simulink model "assemblage_19"  (R2016a)
settings: Solver=ode15s  StartTime=0.0  StopTime=1e6  RelTol=1e-3
undefined symbols (not defined in the file or in its folder): W
libraries: simCryogenics_lib x424, nesl_utility x343, fl_lib x9
(part 3 of 3)

== system assemblage_19/Cryomodules/CMB1 ==
  BP_out-E25 : simCryogenics_lib/Sensors/PTT
  BP_out-E26 : simCryogenics_lib/Sensors/PTT
  Bias25 : Bias  Bias=-50
  Bias26 : Bias  Bias=100
  Constant36 : Constant  Value=W
  Constant37 : Constant  Value=0
  Constant38 : Constant  Value=63
  Distributor19 : simCryogenics_lib/Elements/Distributor2
  FCV00 2 13 : simCryogenics_lib/Elements/Valve  CVmax=0.2  ControlInputMin=0  ControlInputMax=100  Xt=0.86  Rv=100  lin_v=0  lim_v=0  K=2.4e-5 m^1.50000*kg^0.50000/s/bar^0.50000  Cmd_specify=off  Cmd_priority=High  Cmd=0  gamma_specify=off  gamma_priority=High  gamma=0  rho_specify=off  rho_priority=High  rho=0 kg/m^3  Xc_specify=off  Xc_priority=High  Xc=0  X_specify=off  X_priority=High  X=0  Y_specify=off  Y_priority=High  Y=0  CV_specify=off  CV_priority=High  CV=0
  FCV25 : simCryogenics_lib/Elements/Valve  CVmax=1.25  ControlInputMin=0  ControlInputMax=100  Xt=0.86  Rv=150  lin_v=0  lim_v=0  K=2.4e-5 m^1.50000*kg^0.50000/s/bar^0.50000  Cmd_specify=off  Cmd_priority=High  Cmd=0  gamma_specify=off  gamma_priority=High  gamma=0  rho_specify=off  rho_priority=High  rho=0 kg/m^3  Xc_specify=off  Xc_priority=High  Xc=0  X_specify=off  X_priority=High  X=0  Y_specify=off  Y_priority=High  Y=0  CV_specify=off  CV_priority=High  CV=0
  FCV26 : simCryogenics_lib/Elements/Valve  CVmax=1.5  ControlInputMin=0  ControlInputMax=100  Xt=0.86  Rv=100  lin_v=0  lim_v=0  K=2.4e-5 m^1.50000*kg^0.50000/s/bar^0.50000  Cmd_specify=off  Cmd_priority=High  Cmd=0  gamma_specify=off  gamma_priority=High  gamma=0  rho_specify=off  rho_priority=High  rho=0 kg/m^3  Xc_specify=off  Xc_priority=High  Xc=0  X_specify=off  X_priority=High  X=0  Y_specify=off  Y_priority=High  Y=0  CV_specify=off  CV_priority=High  CV=0
  FT73 : simCryogenics_lib/Sensors/FT
  FT74 : Scope
  FT75 : Scope
  FT76 : simCryogenics_lib/Sensors/FT
  FT77 : simCryogenics_lib/Sensors/FT
  FT78 : Scope
  Gain13 : Gain  Gain=-10
  M src37 : simCryogenics_lib/Sources_Sinks/M src  M=0 kg/s
  M src38 : simCryogenics_lib/Sources_Sinks/M src  M=0 kg/s
  M src39 : simCryogenics_lib/Sources_Sinks/M src  M=0 kg/s
  Mixer21 : simCryogenics_lib/Elements/Mixer2
  Mux37 : Mux  Inputs=2
  Mux38 : Mux  Inputs=2
  Mux39 : Mux  Inputs=2
  P/T src25 : simCryogenics_lib/Sources_Sinks/P//T src  P=1.2 bar  T=4.4 K
  P/T src26 : simCryogenics_lib/Sources_Sinks/P//T src  P=1.2 bar  T=4.4 K
  PS-Simulink Converter{133..143} (11 alike) : nesl_utility/PS-Simulink Converter  PhysicalDomain=network_engine_domain  SubClassName=ps_output  LeftPortType=input  RightPortType=output  PseudoPeriodic=off  Frequencies=[]  Unit=1  AffineConversion=off
  PhaseSep13 : simCryogenics_lib/Elements/PhaseSep  Ideal1=1  DeltaT1=0.05 K  N1=10  h1=400 W/K  Ideal2=1  DeltaT2=0.05 K  N2=10  h2=400 W/K  hmax=0.870 m  S=0.0402 m^2  P0=1.25 bar  h0=50  T0=4.5 K
  Simulink-PS Converter{49..52} (4 alike) : nesl_utility/Simulink-PS Converter  PhysicalDomain=network_engine_domain  SubClassName=ps_input  LeftPortType=input  RightPortType=output  PseudoPeriodic=off  Frequencies=[]  NoiseDistribution=none  NoiseParameters=[]  Unit=1  AffineConversion=off  InputFiltering=off  SimscapeFilterOrder=1  InputFilterTimeConstant=0.001  UdotUserProvided=1
  TT49 : Scope
  TT50 : Scope
  TT51 : simCryogenics_lib/Sensors/PTT
  TT52 : Scope
  scope37 : Scope
  scope38 : Scope
  scope39 : Scope
  to_coldbox : PMIOPort  Port=1  Side=Left
  from_dewar : PMIOPort  Port=2  Side=Right
  wires:
  PS-Simulink Converter138/1 -> Mux38/1
  PS-Simulink Converter143/1 -> scope37/1
  Mux38/1 -> TT52/1
  PS-Simulink Converter133/1 -> FT78/1
  Bias26/1 -> scope38/1, Simulink-PS Converter51/1
  Mux37/1 -> TT49/1
  Bias25/1 -> Gain13/1
  Mux39/1 -> TT50/1
  Gain13/1 -> Bias26/1
  PS-Simulink Converter134/1 -> Mux39/1
  PS-Simulink Converter139/1 -> FT75/1
  Constant37/1 -> Simulink-PS Converter50/1
  PS-Simulink Converter137/1 -> FT74/1
  PS-Simulink Converter141/1 -> Mux38/2
  Constant38/1 -> Simulink-PS Converter52/1
  PS-Simulink Converter142/1 -> scope39/1, Bias25/1
  PS-Simulink Converter136/1 -> Mux37/2
  PS-Simulink Converter140/1 -> Mux37/1
  Constant36/1 -> Simulink-PS Converter49/1
  PS-Simulink Converter135/1 -> Mux39/2
  connections:
  Simulink-PS Converter51/RConn1 -- FCV25/LConn1
  BP_out-E26/RConn2 -- PS-Simulink Converter138/LConn1
  FCV26/LConn2 -- PhaseSep13/LConn1 -- BP_out-E25/LConn1 -- FT77/LConn1
  PS-Simulink Converter139/LConn1 -- FT77/RConn1
  PS-Simulink Converter137/LConn1 -- FT73/RConn1
  BP_out-E25/RConn1 -- PS-Simulink Converter135/LConn1
  Simulink-PS Converter50/RConn1 -- FCV00 2 13/LConn1
  PhaseSep13/LConn2 -- P/T src25/RConn1
  from_dewar/RConn1 -- Distributor19/LConn1
  M src37/RConn1 -- PhaseSep13/RConn1
  FCV26/LConn1 -- Simulink-PS Converter52/RConn1
  FCV00 2 13/LConn2 -- Distributor19/RConn1
  PhaseSep13/LConn4 -- Mixer21/RConn1
  FT73/LConn1 -- TT51/LConn1 -- FCV00 2 13/RConn1 -- Mixer21/LConn1
  BP_out-E25/RConn2 -- PS-Simulink Converter134/LConn1
  TT51/RConn1 -- PS-Simulink Converter140/LConn1
  PS-Simulink Converter142/LConn1 -- PhaseSep13/RConn5
  FCV25/RConn1 -- Mixer21/LConn2 -- FT76/LConn1 -- BP_out-E26/LConn1
  PS-Simulink Converter143/LConn1 -- PhaseSep13/LConn5
  M src39/RConn1 -- PhaseSep13/RConn3
  TT51/RConn2 -- PS-Simulink Converter136/LConn1
  FCV26/RConn1 -- to_coldbox/RConn1
  Distributor19/RConn2 -- FCV25/LConn2
  BP_out-E26/RConn1 -- PS-Simulink Converter141/LConn1
  PS-Simulink Converter133/LConn1 -- FT76/RConn1
  PhaseSep13/RConn2 -- M src38/RConn1
  P/T src26/RConn1 -- PhaseSep13/LConn3
  Simulink-PS Converter49/RConn1 -- PhaseSep13/RConn4

== system assemblage_19/Cryomodules/CMB2 ==
  BP_out-E27 : simCryogenics_lib/Sensors/PTT
  BP_out-E28 : simCryogenics_lib/Sensors/PTT
  Bias27 : Bias  Bias=-50
  Bias28 : Bias  Bias=100
  Constant39 : Constant  Value=W
  Constant40 : Constant  Value=0
  Constant41 : Constant  Value=63
  Distributor20 : simCryogenics_lib/Elements/Distributor2
  FCV00 2 14 : simCryogenics_lib/Elements/Valve  CVmax=0.2  ControlInputMin=0  ControlInputMax=100  Xt=0.86  Rv=100  lin_v=0  lim_v=0  K=2.4e-5 m^1.50000*kg^0.50000/s/bar^0.50000  Cmd_specify=off  Cmd_priority=High  Cmd=0  gamma_specify=off  gamma_priority=High  gamma=0  rho_specify=off  rho_priority=High  rho=0 kg/m^3  Xc_specify=off  Xc_priority=High  Xc=0  X_specify=off  X_priority=High  X=0  Y_specify=off  Y_priority=High  Y=0  CV_specify=off  CV_priority=High  CV=0
  FCV27 : simCryogenics_lib/Elements/Valve  CVmax=1.25  ControlInputMin=0  ControlInputMax=100  Xt=0.86  Rv=150  lin_v=0  lim_v=0  K=2.4e-5 m^1.50000*kg^0.50000/s/bar^0.50000  Cmd_specify=off  Cmd_priority=High  Cmd=0  gamma_specify=off  gamma_priority=High  gamma=0  rho_specify=off  rho_priority=High  rho=0 kg/m^3  Xc_specify=off  Xc_priority=High  Xc=0  X_specify=off  X_priority=High  X=0  Y_specify=off  Y_priority=High  Y=0  CV_specify=off  CV_priority=High  CV=0
  FCV28 : simCryogenics_lib/Elements/Valve  CVmax=1.5  ControlInputMin=0  ControlInputMax=100  Xt=0.86  Rv=100  lin_v=0  lim_v=0  K=2.4e-5 m^1.50000*kg^0.50000/s/bar^0.50000  Cmd_specify=off  Cmd_priority=High  Cmd=0  gamma_specify=off  gamma_priority=High  gamma=0  rho_specify=off  rho_priority=High  rho=0 kg/m^3  Xc_specify=off  Xc_priority=High  Xc=0  X_specify=off  X_priority=High  X=0  Y_specify=off  Y_priority=High  Y=0  CV_specify=off  CV_priority=High  CV=0
  FT79 : simCryogenics_lib/Sensors/FT
  FT80 : Scope
  FT81 : Scope
  FT82 : simCryogenics_lib/Sensors/FT
  FT83 : simCryogenics_lib/Sensors/FT
  FT84 : Scope
  Gain14 : Gain  Gain=-10
  M src40 : simCryogenics_lib/Sources_Sinks/M src  M=0 kg/s
  M src41 : simCryogenics_lib/Sources_Sinks/M src  M=0 kg/s
  M src42 : simCryogenics_lib/Sources_Sinks/M src  M=0 kg/s
  Mixer22 : simCryogenics_lib/Elements/Mixer2
  Mux40 : Mux  Inputs=2
  Mux41 : Mux  Inputs=2
  Mux42 : Mux  Inputs=2
  P/T src27 : simCryogenics_lib/Sources_Sinks/P//T src  P=1.2 bar  T=4.4 K
  P/T src28 : simCryogenics_lib/Sources_Sinks/P//T src  P=1.2 bar  T=4.4 K
  PS-Simulink Converter{144..154} (11 alike) : nesl_utility/PS-Simulink Converter  PhysicalDomain=network_engine_domain  SubClassName=ps_output  LeftPortType=input  RightPortType=output  PseudoPeriodic=off  Frequencies=[]  Unit=1  AffineConversion=off
  PhaseSep14 : simCryogenics_lib/Elements/PhaseSep  Ideal1=1  DeltaT1=0.05 K  N1=10  h1=400 W/K  Ideal2=1  DeltaT2=0.05 K  N2=10  h2=400 W/K  hmax=0.870 m  S=0.0402 m^2  P0=1.25 bar  h0=50  T0=4.5 K
  Simulink-PS Converter{53..56} (4 alike) : nesl_utility/Simulink-PS Converter  PhysicalDomain=network_engine_domain  SubClassName=ps_input  LeftPortType=input  RightPortType=output  PseudoPeriodic=off  Frequencies=[]  NoiseDistribution=none  NoiseParameters=[]  Unit=1  AffineConversion=off  InputFiltering=off  SimscapeFilterOrder=1  InputFilterTimeConstant=0.001  UdotUserProvided=1
  TT53 : Scope
  TT54 : Scope
  TT55 : simCryogenics_lib/Sensors/PTT
  TT56 : Scope
  scope40 : Scope
  scope41 : Scope
  scope42 : Scope
  to_coldbox : PMIOPort  Port=1  Side=Left
  from_dewar : PMIOPort  Port=2  Side=Right
  wires:
  PS-Simulink Converter149/1 -> Mux41/1
  PS-Simulink Converter148/1 -> FT80/1
  Mux40/1 -> TT53/1
  PS-Simulink Converter151/1 -> Mux40/1
  Bias28/1 -> scope41/1, Simulink-PS Converter55/1
  PS-Simulink Converter147/1 -> Mux40/2
  Constant40/1 -> Simulink-PS Converter54/1
  PS-Simulink Converter145/1 -> Mux42/1
  Constant39/1 -> Simulink-PS Converter53/1
  PS-Simulink Converter150/1 -> FT81/1
  Mux42/1 -> TT54/1
  Gain14/1 -> Bias28/1
  PS-Simulink Converter144/1 -> FT84/1
  PS-Simulink Converter146/1 -> Mux42/2
  Bias27/1 -> Gain14/1
  Constant41/1 -> Simulink-PS Converter56/1
  PS-Simulink Converter152/1 -> Mux41/2
  PS-Simulink Converter154/1 -> scope40/1
  Mux41/1 -> TT56/1
  PS-Simulink Converter153/1 -> scope42/1, Bias27/1
  connections:
  FCV28/LConn2 -- PhaseSep14/LConn1 -- BP_out-E27/LConn1 -- FT83/LConn1
  FT79/LConn1 -- TT55/LConn1 -- FCV00 2 14/RConn1 -- Mixer22/LConn1
  BP_out-E27/RConn1 -- PS-Simulink Converter146/LConn1
  Distributor20/RConn2 -- FCV27/LConn2
  PS-Simulink Converter154/LConn1 -- PhaseSep14/LConn5
  BP_out-E28/RConn1 -- PS-Simulink Converter152/LConn1
  Simulink-PS Converter54/RConn1 -- FCV00 2 14/LConn1
  PhaseSep14/RConn2 -- M src41/RConn1
  TT55/RConn1 -- PS-Simulink Converter151/LConn1
  BP_out-E28/RConn2 -- PS-Simulink Converter149/LConn1
  FCV28/LConn1 -- Simulink-PS Converter56/RConn1
  PS-Simulink Converter153/LConn1 -- PhaseSep14/RConn5
  from_dewar/RConn1 -- Distributor20/LConn1
  M src42/RConn1 -- PhaseSep14/RConn3
  TT55/RConn2 -- PS-Simulink Converter147/LConn1
  PhaseSep14/LConn2 -- P/T src27/RConn1
  FCV28/RConn1 -- to_coldbox/RConn1
  P/T src28/RConn1 -- PhaseSep14/LConn3
  BP_out-E27/RConn2 -- PS-Simulink Converter145/LConn1
  FCV00 2 14/LConn2 -- Distributor20/RConn1
  PS-Simulink Converter144/LConn1 -- FT82/RConn1
  Simulink-PS Converter53/RConn1 -- PhaseSep14/RConn4
  Simulink-PS Converter55/RConn1 -- FCV27/LConn1
  PS-Simulink Converter148/LConn1 -- FT79/RConn1
  PhaseSep14/LConn4 -- Mixer22/RConn1
  PS-Simulink Converter150/LConn1 -- FT83/RConn1
  FCV27/RConn1 -- Mixer22/LConn2 -- FT82/LConn1 -- BP_out-E28/LConn1
  M src40/RConn1 -- PhaseSep14/RConn1

== system assemblage_19/Cryomodules/CMB3 ==
  BP_out-E29 : simCryogenics_lib/Sensors/PTT
  BP_out-E30 : simCryogenics_lib/Sensors/PTT
  Bias29 : Bias  Bias=-50
  Bias30 : Bias  Bias=100
  Constant42 : Constant  Value=W
  Constant43 : Constant  Value=0
  Constant44 : Constant  Value=63
  Distributor21 : simCryogenics_lib/Elements/Distributor2
  FCV00 2 15 : simCryogenics_lib/Elements/Valve  CVmax=0.2  ControlInputMin=0  ControlInputMax=100  Xt=0.86  Rv=100  lin_v=0  lim_v=0  K=2.4e-5 m^1.50000*kg^0.50000/s/bar^0.50000  Cmd_specify=off  Cmd_priority=High  Cmd=0  gamma_specify=off  gamma_priority=High  gamma=0  rho_specify=off  rho_priority=High  rho=0 kg/m^3  Xc_specify=off  Xc_priority=High  Xc=0  X_specify=off  X_priority=High  X=0  Y_specify=off  Y_priority=High  Y=0  CV_specify=off  CV_priority=High  CV=0
  FCV29 : simCryogenics_lib/Elements/Valve  CVmax=1.25  ControlInputMin=0  ControlInputMax=100  Xt=0.86  Rv=150  lin_v=0  lim_v=0  K=2.4e-5 m^1.50000*kg^0.50000/s/bar^0.50000  Cmd_specify=off  Cmd_priority=High  Cmd=0  gamma_specify=off  gamma_priority=High  gamma=0  rho_specify=off  rho_priority=High  rho=0 kg/m^3  Xc_specify=off  Xc_priority=High  Xc=0  X_specify=off  X_priority=High  X=0  Y_specify=off  Y_priority=High  Y=0  CV_specify=off  CV_priority=High  CV=0
  FCV30 : simCryogenics_lib/Elements/Valve  CVmax=1.5  ControlInputMin=0  ControlInputMax=100  Xt=0.86  Rv=100  lin_v=0  lim_v=0  K=2.4e-5 m^1.50000*kg^0.50000/s/bar^0.50000  Cmd_specify=off  Cmd_priority=High  Cmd=0  gamma_specify=off  gamma_priority=High  gamma=0  rho_specify=off  rho_priority=High  rho=0 kg/m^3  Xc_specify=off  Xc_priority=High  Xc=0  X_specify=off  X_priority=High  X=0  Y_specify=off  Y_priority=High  Y=0  CV_specify=off  CV_priority=High  CV=0
  FT85 : simCryogenics_lib/Sensors/FT
  FT86 : Scope
  FT87 : Scope
  FT88 : simCryogenics_lib/Sensors/FT
  FT89 : simCryogenics_lib/Sensors/FT
  FT90 : Scope
  Gain15 : Gain  Gain=-10
  M src43 : simCryogenics_lib/Sources_Sinks/M src  M=0 kg/s
  M src44 : simCryogenics_lib/Sources_Sinks/M src  M=0 kg/s
  M src45 : simCryogenics_lib/Sources_Sinks/M src  M=0 kg/s
  Mixer23 : simCryogenics_lib/Elements/Mixer2
  Mux43 : Mux  Inputs=2
  Mux44 : Mux  Inputs=2
  Mux45 : Mux  Inputs=2
  P/T src29 : simCryogenics_lib/Sources_Sinks/P//T src  P=1.2 bar  T=4.4 K
  P/T src30 : simCryogenics_lib/Sources_Sinks/P//T src  P=1.2 bar  T=4.4 K
  PS-Simulink Converter{155..165} (11 alike) : nesl_utility/PS-Simulink Converter  PhysicalDomain=network_engine_domain  SubClassName=ps_output  LeftPortType=input  RightPortType=output  PseudoPeriodic=off  Frequencies=[]  Unit=1  AffineConversion=off
  PhaseSep15 : simCryogenics_lib/Elements/PhaseSep  Ideal1=1  DeltaT1=0.05 K  N1=10  h1=400 W/K  Ideal2=1  DeltaT2=0.05 K  N2=10  h2=400 W/K  hmax=0.870 m  S=0.0402 m^2  P0=1.25 bar  h0=50  T0=4.5 K
  Simulink-PS Converter{57..60} (4 alike) : nesl_utility/Simulink-PS Converter  PhysicalDomain=network_engine_domain  SubClassName=ps_input  LeftPortType=input  RightPortType=output  PseudoPeriodic=off  Frequencies=[]  NoiseDistribution=none  NoiseParameters=[]  Unit=1  AffineConversion=off  InputFiltering=off  SimscapeFilterOrder=1  InputFilterTimeConstant=0.001  UdotUserProvided=1
  TT57 : Scope
  TT58 : Scope
  TT59 : simCryogenics_lib/Sensors/PTT
  TT60 : Scope
  scope43 : Scope
  scope44 : Scope
  scope45 : Scope
  to_coldbox : PMIOPort  Port=1  Side=Left
  from_dewar : PMIOPort  Port=2  Side=Right
  wires:
  Bias29/1 -> Gain15/1
  PS-Simulink Converter160/1 -> Mux44/1
  Constant43/1 -> Simulink-PS Converter58/1
  PS-Simulink Converter161/1 -> FT87/1
  PS-Simulink Converter157/1 -> Mux45/2
  Constant42/1 -> Simulink-PS Converter57/1
  PS-Simulink Converter159/1 -> FT86/1
  Mux44/1 -> TT60/1
  PS-Simulink Converter164/1 -> scope45/1, Bias29/1
  PS-Simulink Converter163/1 -> Mux44/2
  Constant44/1 -> Simulink-PS Converter60/1
  Gain15/1 -> Bias30/1
  PS-Simulink Converter155/1 -> FT90/1
  PS-Simulink Converter165/1 -> scope43/1
  PS-Simulink Converter156/1 -> Mux45/1
  Mux43/1 -> TT57/1
  PS-Simulink Converter162/1 -> Mux43/1
  Bias30/1 -> scope44/1, Simulink-PS Converter59/1
  Mux45/1 -> TT58/1
  PS-Simulink Converter158/1 -> Mux43/2
  connections:
  PS-Simulink Converter155/LConn1 -- FT88/RConn1
  FT85/LConn1 -- TT59/LConn1 -- FCV00 2 15/RConn1 -- Mixer23/LConn1
  BP_out-E29/RConn2 -- PS-Simulink Converter156/LConn1
  P/T src30/RConn1 -- PhaseSep15/LConn3
  PS-Simulink Converter159/LConn1 -- FT85/RConn1
  M src43/RConn1 -- PhaseSep15/RConn1
  M src45/RConn1 -- PhaseSep15/RConn3
  BP_out-E30/RConn1 -- PS-Simulink Converter163/LConn1
  BP_out-E30/RConn2 -- PS-Simulink Converter160/LConn1
  PS-Simulink Converter164/LConn1 -- PhaseSep15/RConn5
  PS-Simulink Converter165/LConn1 -- PhaseSep15/LConn5
  BP_out-E29/RConn1 -- PS-Simulink Converter157/LConn1
  from_dewar/RConn1 -- Distributor21/LConn1
  PhaseSep15/LConn4 -- Mixer23/RConn1
  TT59/RConn1 -- PS-Simulink Converter162/LConn1
  FCV00 2 15/LConn2 -- Distributor21/RConn1
  Simulink-PS Converter58/RConn1 -- FCV00 2 15/LConn1
  PhaseSep15/RConn2 -- M src44/RConn1
  Simulink-PS Converter59/RConn1 -- FCV29/LConn1
  Distributor21/RConn2 -- FCV29/LConn2
  TT59/RConn2 -- PS-Simulink Converter158/LConn1
  FCV29/RConn1 -- Mixer23/LConn2 -- FT88/LConn1 -- BP_out-E30/LConn1
  PS-Simulink Converter161/LConn1 -- FT89/RConn1
  Simulink-PS Converter57/RConn1 -- PhaseSep15/RConn4
  FCV30/RConn1 -- to_coldbox/RConn1
  PhaseSep15/LConn2 -- P/T src29/RConn1
  FCV30/LConn2 -- PhaseSep15/LConn1 -- BP_out-E29/LConn1 -- FT89/LConn1
  FCV30/LConn1 -- Simulink-PS Converter60/RConn1

== system assemblage_19/Cryomodules/CMB4 ==
  BP_out-E31 : simCryogenics_lib/Sensors/PTT
  BP_out-E32 : simCryogenics_lib/Sensors/PTT
  Bias31 : Bias  Bias=-50
  Bias32 : Bias  Bias=100
  Constant45 : Constant  Value=W
  Constant46 : Constant  Value=0
  Constant47 : Constant  Value=63
  Distributor22 : simCryogenics_lib/Elements/Distributor2
  FCV00 2 16 : simCryogenics_lib/Elements/Valve  CVmax=0.2  ControlInputMin=0  ControlInputMax=100  Xt=0.86  Rv=100  lin_v=0  lim_v=0  K=2.4e-5 m^1.50000*kg^0.50000/s/bar^0.50000  Cmd_specify=off  Cmd_priority=High  Cmd=0  gamma_specify=off  gamma_priority=High  gamma=0  rho_specify=off  rho_priority=High  rho=0 kg/m^3  Xc_specify=off  Xc_priority=High  Xc=0  X_specify=off  X_priority=High  X=0  Y_specify=off  Y_priority=High  Y=0  CV_specify=off  CV_priority=High  CV=0
  FCV31 : simCryogenics_lib/Elements/Valve  CVmax=1.25  ControlInputMin=0  ControlInputMax=100  Xt=0.86  Rv=150  lin_v=0  lim_v=0  K=2.4e-5 m^1.50000*kg^0.50000/s/bar^0.50000  Cmd_specify=off  Cmd_priority=High  Cmd=0  gamma_specify=off  gamma_priority=High  gamma=0  rho_specify=off  rho_priority=High  rho=0 kg/m^3  Xc_specify=off  Xc_priority=High  Xc=0  X_specify=off  X_priority=High  X=0  Y_specify=off  Y_priority=High  Y=0  CV_specify=off  CV_priority=High  CV=0
  FCV32 : simCryogenics_lib/Elements/Valve  CVmax=1.5  ControlInputMin=0  ControlInputMax=100  Xt=0.86  Rv=100  lin_v=0  lim_v=0  K=2.4e-5 m^1.50000*kg^0.50000/s/bar^0.50000  Cmd_specify=off  Cmd_priority=High  Cmd=0  gamma_specify=off  gamma_priority=High  gamma=0  rho_specify=off  rho_priority=High  rho=0 kg/m^3  Xc_specify=off  Xc_priority=High  Xc=0  X_specify=off  X_priority=High  X=0  Y_specify=off  Y_priority=High  Y=0  CV_specify=off  CV_priority=High  CV=0
  FT91 : simCryogenics_lib/Sensors/FT
  FT92 : Scope
  FT93 : Scope
  FT94 : simCryogenics_lib/Sensors/FT
  FT95 : simCryogenics_lib/Sensors/FT
  FT96 : Scope
  Gain16 : Gain  Gain=-10
  M src46 : simCryogenics_lib/Sources_Sinks/M src  M=0 kg/s
  M src47 : simCryogenics_lib/Sources_Sinks/M src  M=0 kg/s
  M src48 : simCryogenics_lib/Sources_Sinks/M src  M=0 kg/s
  Mixer24 : simCryogenics_lib/Elements/Mixer2
  Mux46 : Mux  Inputs=2
  Mux47 : Mux  Inputs=2
  Mux48 : Mux  Inputs=2
  P/T src31 : simCryogenics_lib/Sources_Sinks/P//T src  P=1.2 bar  T=4.4 K
  P/T src32 : simCryogenics_lib/Sources_Sinks/P//T src  P=1.2 bar  T=4.4 K
  PS-Simulink Converter{166..176} (11 alike) : nesl_utility/PS-Simulink Converter  PhysicalDomain=network_engine_domain  SubClassName=ps_output  LeftPortType=input  RightPortType=output  PseudoPeriodic=off  Frequencies=[]  Unit=1  AffineConversion=off
  PhaseSep16 : simCryogenics_lib/Elements/PhaseSep  Ideal1=1  DeltaT1=0.05 K  N1=10  h1=400 W/K  Ideal2=1  DeltaT2=0.05 K  N2=10  h2=400 W/K  hmax=0.870 m  S=0.0402 m^2  P0=1.25 bar  h0=50  T0=4.5 K
  Simulink-PS Converter{61..64} (4 alike) : nesl_utility/Simulink-PS Converter  PhysicalDomain=network_engine_domain  SubClassName=ps_input  LeftPortType=input  RightPortType=output  PseudoPeriodic=off  Frequencies=[]  NoiseDistribution=none  NoiseParameters=[]  Unit=1  AffineConversion=off  InputFiltering=off  SimscapeFilterOrder=1  InputFilterTimeConstant=0.001  UdotUserProvided=1
  TT61 : Scope
  TT62 : Scope
  TT63 : simCryogenics_lib/Sensors/PTT
  TT64 : Scope
  scope46 : Scope
  scope47 : Scope
  scope48 : Scope
  to_coldbox : PMIOPort  Port=1  Side=Left
  from_dewar : PMIOPort  Port=2  Side=Right
  wires:
  Gain16/1 -> Bias32/1
  PS-Simulink Converter173/1 -> Mux46/1
  PS-Simulink Converter166/1 -> FT96/1
  PS-Simulink Converter169/1 -> Mux46/2
  PS-Simulink Converter170/1 -> FT92/1
  Constant47/1 -> Simulink-PS Converter64/1
  PS-Simulink Converter171/1 -> Mux47/1
  PS-Simulink Converter176/1 -> scope46/1
  PS-Simulink Converter175/1 -> scope48/1, Bias31/1
  Mux48/1 -> TT62/1
  PS-Simulink Converter168/1 -> Mux48/2
  Constant45/1 -> Simulink-PS Converter61/1
  PS-Simulink Converter174/1 -> Mux47/2
  Bias31/1 -> Gain16/1
  Bias32/1 -> scope47/1, Simulink-PS Converter63/1
  PS-Simulink Converter167/1 -> Mux48/1
  Mux46/1 -> TT61/1
  Constant46/1 -> Simulink-PS Converter62/1
  PS-Simulink Converter172/1 -> FT93/1
  Mux47/1 -> TT64/1
  connections:
  PS-Simulink Converter170/LConn1 -- FT91/RConn1
  PS-Simulink Converter176/LConn1 -- PhaseSep16/LConn5
  Simulink-PS Converter61/RConn1 -- PhaseSep16/RConn4
  PS-Simulink Converter175/LConn1 -- PhaseSep16/RConn5
  BP_out-E31/RConn2 -- PS-Simulink Converter167/LConn1
  M src48/RConn1 -- PhaseSep16/RConn3
  P/T src32/RConn1 -- PhaseSep16/LConn3
  PhaseSep16/LConn4 -- Mixer24/RConn1
  PhaseSep16/LConn2 -- P/T src31/RConn1
  FT91/LConn1 -- TT63/LConn1 -- FCV00 2 16/RConn1 -- Mixer24/LConn1
  BP_out-E31/RConn1 -- PS-Simulink Converter168/LConn1
  Simulink-PS Converter62/RConn1 -- FCV00 2 16/LConn1
  BP_out-E32/RConn1 -- PS-Simulink Converter174/LConn1
  M src46/RConn1 -- PhaseSep16/RConn1
  TT63/RConn1 -- PS-Simulink Converter173/LConn1
  FCV32/LConn1 -- Simulink-PS Converter64/RConn1
  FCV31/RConn1 -- Mixer24/LConn2 -- FT94/LConn1 -- BP_out-E32/LConn1
  FCV32/RConn1 -- to_coldbox/RConn1
  FCV00 2 16/LConn2 -- Distributor22/RConn1
  PS-Simulink Converter172/LConn1 -- FT95/RConn1
  PS-Simulink Converter166/LConn1 -- FT94/RConn1
  Simulink-PS Converter63/RConn1 -- FCV31/LConn1
  PhaseSep16/RConn2 -- M src47/RConn1
  Distributor22/RConn2 -- FCV31/LConn2
  from_dewar/RConn1 -- Distributor22/LConn1
  TT63/RConn2 -- PS-Simulink Converter169/LConn1
  FCV32/LConn2 -- PhaseSep16/LConn1 -- BP_out-E31/LConn1 -- FT95/LConn1
  BP_out-E32/RConn2 -- PS-Simulink Converter171/LConn1

== system assemblage_19/Cryomodules/CMB5 ==
  BP_out-E33 : simCryogenics_lib/Sensors/PTT
  BP_out-E34 : simCryogenics_lib/Sensors/PTT
  Bias33 : Bias  Bias=-50
  Bias34 : Bias  Bias=100
  Constant48 : Constant  Value=W
  Constant49 : Constant  Value=0
  Constant50 : Constant  Value=63
  Distributor23 : simCryogenics_lib/Elements/Distributor2
  FCV00 2 17 : simCryogenics_lib/Elements/Valve  CVmax=0.2  ControlInputMin=0  ControlInputMax=100  Xt=0.86  Rv=100  lin_v=0  lim_v=0  K=2.4e-5 m^1.50000*kg^0.50000/s/bar^0.50000  Cmd_specify=off  Cmd_priority=High  Cmd=0  gamma_specify=off  gamma_priority=High  gamma=0  rho_specify=off  rho_priority=High  rho=0 kg/m^3  Xc_specify=off  Xc_priority=High  Xc=0  X_specify=off  X_priority=High  X=0  Y_specify=off  Y_priority=High  Y=0  CV_specify=off  CV_priority=High  CV=0
  FCV33 : simCryogenics_lib/Elements/Valve  CVmax=1.25  ControlInputMin=0  ControlInputMax=100  Xt=0.86  Rv=150  lin_v=0  lim_v=0  K=2.4e-5 m^1.50000*kg^0.50000/s/bar^0.50000  Cmd_specify=off  Cmd_priority=High  Cmd=0  gamma_specify=off  gamma_priority=High  gamma=0  rho_specify=off  rho_priority=High  rho=0 kg/m^3  Xc_specify=off  Xc_priority=High  Xc=0  X_specify=off  X_priority=High  X=0  Y_specify=off  Y_priority=High  Y=0  CV_specify=off  CV_priority=High  CV=0
  FCV34 : simCryogenics_lib/Elements/Valve  CVmax=1.5  ControlInputMin=0  ControlInputMax=100  Xt=0.86  Rv=100  lin_v=0  lim_v=0  K=2.4e-5 m^1.50000*kg^0.50000/s/bar^0.50000  Cmd_specify=off  Cmd_priority=High  Cmd=0  gamma_specify=off  gamma_priority=High  gamma=0  rho_specify=off  rho_priority=High  rho=0 kg/m^3  Xc_specify=off  Xc_priority=High  Xc=0  X_specify=off  X_priority=High  X=0  Y_specify=off  Y_priority=High  Y=0  CV_specify=off  CV_priority=High  CV=0
  FT100 : simCryogenics_lib/Sensors/FT
  FT101 : simCryogenics_lib/Sensors/FT
  FT102 : Scope
  FT97 : simCryogenics_lib/Sensors/FT
  FT98 : Scope
  FT99 : Scope
  Gain17 : Gain  Gain=-10
  M src49 : simCryogenics_lib/Sources_Sinks/M src  M=0 kg/s
  M src50 : simCryogenics_lib/Sources_Sinks/M src  M=0 kg/s
  M src51 : simCryogenics_lib/Sources_Sinks/M src  M=0 kg/s
  Mixer25 : simCryogenics_lib/Elements/Mixer2
  Mux49 : Mux  Inputs=2
  Mux50 : Mux  Inputs=2
  Mux51 : Mux  Inputs=2
  P/T src33 : simCryogenics_lib/Sources_Sinks/P//T src  P=1.2 bar  T=4.4 K
  P/T src34 : simCryogenics_lib/Sources_Sinks/P//T src  P=1.2 bar  T=4.4 K
  PS-Simulink Converter{177..187} (11 alike) : nesl_utility/PS-Simulink Converter  PhysicalDomain=network_engine_domain  SubClassName=ps_output  LeftPortType=input  RightPortType=output  PseudoPeriodic=off  Frequencies=[]  Unit=1  AffineConversion=off
  PhaseSep17 : simCryogenics_lib/Elements/PhaseSep  Ideal1=1  DeltaT1=0.05 K  N1=10  h1=400 W/K  Ideal2=1  DeltaT2=0.05 K  N2=10  h2=400 W/K  hmax=0.870 m  S=0.0402 m^2  P0=1.25 bar  h0=50  T0=4.5 K
  Simulink-PS Converter{65..68} (4 alike) : nesl_utility/Simulink-PS Converter  PhysicalDomain=network_engine_domain  SubClassName=ps_input  LeftPortType=input  RightPortType=output  PseudoPeriodic=off  Frequencies=[]  NoiseDistribution=none  NoiseParameters=[]  Unit=1  AffineConversion=off  InputFiltering=off  SimscapeFilterOrder=1  InputFilterTimeConstant=0.001  UdotUserProvided=1
  TT65 : Scope
  TT66 : Scope
  TT67 : simCryogenics_lib/Sensors/PTT
  TT68 : Scope
  scope49 : Scope
  scope50 : Scope
  scope51 : Scope
  to_coldbox : PMIOPort  Port=1  Side=Left
  from_dewar : PMIOPort  Port=2  Side=Right
  wires:
  PS-Simulink Converter186/1 -> scope51/1, Bias33/1
  PS-Simulink Converter187/1 -> scope49/1
  PS-Simulink Converter183/1 -> FT99/1
  Bias33/1 -> Gain17/1
  PS-Simulink Converter181/1 -> FT98/1
  Gain17/1 -> Bias34/1
  Constant49/1 -> Simulink-PS Converter66/1
  Mux50/1 -> TT68/1
  Mux51/1 -> TT66/1
  Constant50/1 -> Simulink-PS Converter68/1
  PS-Simulink Converter182/1 -> Mux50/1
  PS-Simulink Converter178/1 -> Mux51/1
  Constant48/1 -> Simulink-PS Converter65/1
  PS-Simulink Converter184/1 -> Mux49/1
  PS-Simulink Converter185/1 -> Mux50/2
  PS-Simulink Converter180/1 -> Mux49/2
  Bias34/1 -> scope50/1, Simulink-PS Converter67/1
  Mux49/1 -> TT65/1
  PS-Simulink Converter177/1 -> FT102/1
  PS-Simulink Converter179/1 -> Mux51/2
  connections:
  PhaseSep17/LConn2 -- P/T src33/RConn1
  FCV34/LConn1 -- Simulink-PS Converter68/RConn1
  FCV00 2 17/LConn2 -- Distributor23/RConn1
  Simulink-PS Converter67/RConn1 -- FCV33/LConn1
  PhaseSep17/LConn4 -- Mixer25/RConn1
  PS-Simulink Converter181/LConn1 -- FT97/RConn1
  Simulink-PS Converter65/RConn1 -- PhaseSep17/RConn4
  PS-Simulink Converter183/LConn1 -- FT101/RConn1
  M src49/RConn1 -- PhaseSep17/RConn1
  Simulink-PS Converter66/RConn1 -- FCV00 2 17/LConn1
  PhaseSep17/RConn2 -- M src50/RConn1
  BP_out-E34/RConn2 -- PS-Simulink Converter182/LConn1
  PS-Simulink Converter187/LConn1 -- PhaseSep17/LConn5
  M src51/RConn1 -- PhaseSep17/RConn3
  BP_out-E33/RConn1 -- PS-Simulink Converter179/LConn1
  PS-Simulink Converter186/LConn1 -- PhaseSep17/RConn5
  FCV34/LConn2 -- PhaseSep17/LConn1 -- BP_out-E33/LConn1 -- FT101/LConn1
  FCV34/RConn1 -- to_coldbox/RConn1
  PS-Simulink Converter177/LConn1 -- FT100/RConn1
  BP_out-E33/RConn2 -- PS-Simulink Converter178/LConn1
  BP_out-E34/RConn1 -- PS-Simulink Converter185/LConn1
  TT67/RConn2 -- PS-Simulink Converter180/LConn1
  P/T src34/RConn1 -- PhaseSep17/LConn3
  TT67/RConn1 -- PS-Simulink Converter184/LConn1
  from_dewar/RConn1 -- Distributor23/LConn1
  Distributor23/RConn2 -- FCV33/LConn2
  FT97/LConn1 -- TT67/LConn1 -- FCV00 2 17/RConn1 -- Mixer25/LConn1
  FCV33/RConn1 -- Mixer25/LConn2 -- FT100/LConn1 -- BP_out-E34/LConn1

== system assemblage_19/Cryomodules/CMB6 ==
  BP_out-E35 : simCryogenics_lib/Sensors/PTT
  BP_out-E36 : simCryogenics_lib/Sensors/PTT
  Bias35 : Bias  Bias=-50
  Bias36 : Bias  Bias=100
  Constant51 : Constant  Value=W
  Constant52 : Constant  Value=0
  Constant53 : Constant  Value=63
  Distributor24 : simCryogenics_lib/Elements/Distributor2
  FCV00 2 18 : simCryogenics_lib/Elements/Valve  CVmax=0.2  ControlInputMin=0  ControlInputMax=100  Xt=0.86  Rv=100  lin_v=0  lim_v=0  K=2.4e-5 m^1.50000*kg^0.50000/s/bar^0.50000  Cmd_specify=off  Cmd_priority=High  Cmd=0  gamma_specify=off  gamma_priority=High  gamma=0  rho_specify=off  rho_priority=High  rho=0 kg/m^3  Xc_specify=off  Xc_priority=High  Xc=0  X_specify=off  X_priority=High  X=0  Y_specify=off  Y_priority=High  Y=0  CV_specify=off  CV_priority=High  CV=0
  FCV35 : simCryogenics_lib/Elements/Valve  CVmax=1.25  ControlInputMin=0  ControlInputMax=100  Xt=0.86  Rv=150  lin_v=0  lim_v=0  K=2.4e-5 m^1.50000*kg^0.50000/s/bar^0.50000  Cmd_specify=off  Cmd_priority=High  Cmd=0  gamma_specify=off  gamma_priority=High  gamma=0  rho_specify=off  rho_priority=High  rho=0 kg/m^3  Xc_specify=off  Xc_priority=High  Xc=0  X_specify=off  X_priority=High  X=0  Y_specify=off  Y_priority=High  Y=0  CV_specify=off  CV_priority=High  CV=0
  FCV36 : simCryogenics_lib/Elements/Valve  CVmax=1.5  ControlInputMin=0  ControlInputMax=100  Xt=0.86  Rv=100  lin_v=0  lim_v=0  K=2.4e-5 m^1.50000*kg^0.50000/s/bar^0.50000  Cmd_specify=off  Cmd_priority=High  Cmd=0  gamma_specify=off  gamma_priority=High  gamma=0  rho_specify=off  rho_priority=High  rho=0 kg/m^3  Xc_specify=off  Xc_priority=High  Xc=0  X_specify=off  X_priority=High  X=0  Y_specify=off  Y_priority=High  Y=0  CV_specify=off  CV_priority=High  CV=0
  FT103 : simCryogenics_lib/Sensors/FT
  FT104 : Scope
  FT105 : Scope
  FT106 : simCryogenics_lib/Sensors/FT
  FT107 : simCryogenics_lib/Sensors/FT
  FT108 : Scope
  Gain18 : Gain  Gain=-10
  M src52 : simCryogenics_lib/Sources_Sinks/M src  M=0 kg/s
  M src53 : simCryogenics_lib/Sources_Sinks/M src  M=0 kg/s
  M src54 : simCryogenics_lib/Sources_Sinks/M src  M=0 kg/s
  Mixer26 : simCryogenics_lib/Elements/Mixer2
  Mux52 : Mux  Inputs=2
  Mux53 : Mux  Inputs=2
  Mux54 : Mux  Inputs=2
  P/T src35 : simCryogenics_lib/Sources_Sinks/P//T src  P=1.2 bar  T=4.4 K
  P/T src36 : simCryogenics_lib/Sources_Sinks/P//T src  P=1.2 bar  T=4.4 K
  PS-Simulink Converter{188..198} (11 alike) : nesl_utility/PS-Simulink Converter  PhysicalDomain=network_engine_domain  SubClassName=ps_output  LeftPortType=input  RightPortType=output  PseudoPeriodic=off  Frequencies=[]  Unit=1  AffineConversion=off
  PhaseSep18 : simCryogenics_lib/Elements/PhaseSep  Ideal1=1  DeltaT1=0.05 K  N1=10  h1=400 W/K  Ideal2=1  DeltaT2=0.05 K  N2=10  h2=400 W/K  hmax=0.870 m  S=0.0402 m^2  P0=1.25 bar  h0=50  T0=4.5 K
  Simulink-PS Converter{69..72} (4 alike) : nesl_utility/Simulink-PS Converter  PhysicalDomain=network_engine_domain  SubClassName=ps_input  LeftPortType=input  RightPortType=output  PseudoPeriodic=off  Frequencies=[]  NoiseDistribution=none  NoiseParameters=[]  Unit=1  AffineConversion=off  InputFiltering=off  SimscapeFilterOrder=1  InputFilterTimeConstant=0.001  UdotUserProvided=1
  TT69 : Scope
  TT70 : Scope
  TT71 : simCryogenics_lib/Sensors/PTT
  TT72 : Scope
  scope52 : Scope
  scope53 : Scope
  scope54 : Scope
  to_coldbox : PMIOPort  Port=1  Side=Left
  from_dewar : PMIOPort  Port=2  Side=Right
  wires:
  Mux52/1 -> TT69/1
  PS-Simulink Converter198/1 -> scope52/1
  PS-Simulink Converter196/1 -> Mux53/2
  PS-Simulink Converter189/1 -> Mux54/1
  Bias36/1 -> scope53/1, Simulink-PS Converter71/1
  Gain18/1 -> Bias36/1
  PS-Simulink Converter190/1 -> Mux54/2
  Constant53/1 -> Simulink-PS Converter72/1
  PS-Simulink Converter191/1 -> Mux52/2
  PS-Simulink Converter195/1 -> Mux52/1
  Bias35/1 -> Gain18/1
  PS-Simulink Converter197/1 -> scope54/1, Bias35/1
  PS-Simulink Converter193/1 -> Mux53/1
  PS-Simulink Converter194/1 -> FT105/1
  Constant51/1 -> Simulink-PS Converter69/1
  Mux54/1 -> TT70/1
  Mux53/1 -> TT72/1
  PS-Simulink Converter192/1 -> FT104/1
  PS-Simulink Converter188/1 -> FT108/1
  Constant52/1 -> Simulink-PS Converter70/1
  connections:
  FCV36/RConn1 -- to_coldbox/RConn1
  FCV36/LConn1 -- Simulink-PS Converter72/RConn1
  PS-Simulink Converter198/LConn1 -- PhaseSep18/LConn5
  Distributor24/RConn2 -- FCV35/LConn2
  P/T src36/RConn1 -- PhaseSep18/LConn3
  TT71/RConn2 -- PS-Simulink Converter191/LConn1
  FCV00 2 18/LConn2 -- Distributor24/RConn1
  PS-Simulink Converter197/LConn1 -- PhaseSep18/RConn5
  Simulink-PS Converter70/RConn1 -- FCV00 2 18/LConn1
  BP_out-E36/RConn2 -- PS-Simulink Converter193/LConn1
  PS-Simulink Converter188/LConn1 -- FT106/RConn1
  PhaseSep18/RConn2 -- M src53/RConn1
  PS-Simulink Converter192/LConn1 -- FT103/RConn1
  Simulink-PS Converter71/RConn1 -- FCV35/LConn1
  PS-Simulink Converter194/LConn1 -- FT107/RConn1
  FCV36/LConn2 -- PhaseSep18/LConn1 -- BP_out-E35/LConn1 -- FT107/LConn1
  M src52/RConn1 -- PhaseSep18/RConn1
  from_dewar/RConn1 -- Distributor24/LConn1
  M src54/RConn1 -- PhaseSep18/RConn3
  PhaseSep18/LConn2 -- P/T src35/RConn1
  BP_out-E36/RConn1 -- PS-Simulink Converter196/LConn1
  BP_out-E35/RConn1 -- PS-Simulink Converter190/LConn1
  TT71/RConn1 -- PS-Simulink Converter195/LConn1
  FCV35/RConn1 -- Mixer26/LConn2 -- FT106/LConn1 -- BP_out-E36/LConn1
  Simulink-PS Converter69/RConn1 -- PhaseSep18/RConn4
  FT103/LConn1 -- TT71/LConn1 -- FCV00 2 18/RConn1 -- Mixer26/LConn1
  PhaseSep18/LConn4 -- Mixer26/RConn1
  BP_out-E35/RConn2 -- PS-Simulink Converter189/LConn1

== system assemblage_19/Cryomodules/CMB7 ==
  BP_out-E37 : simCryogenics_lib/Sensors/PTT
  BP_out-E38 : simCryogenics_lib/Sensors/PTT
  Bias37 : Bias  Bias=-50
  Bias38 : Bias  Bias=100
  Constant54 : Constant  Value=W
  Constant55 : Constant  Value=0
  Constant56 : Constant  Value=63
  Distributor25 : simCryogenics_lib/Elements/Distributor2
  FCV00 2 19 : simCryogenics_lib/Elements/Valve  CVmax=0.2  ControlInputMin=0  ControlInputMax=100  Xt=0.86  Rv=100  lin_v=0  lim_v=0  K=2.4e-5 m^1.50000*kg^0.50000/s/bar^0.50000  Cmd_specify=off  Cmd_priority=High  Cmd=0  gamma_specify=off  gamma_priority=High  gamma=0  rho_specify=off  rho_priority=High  rho=0 kg/m^3  Xc_specify=off  Xc_priority=High  Xc=0  X_specify=off  X_priority=High  X=0  Y_specify=off  Y_priority=High  Y=0  CV_specify=off  CV_priority=High  CV=0
  FCV37 : simCryogenics_lib/Elements/Valve  CVmax=1.25  ControlInputMin=0  ControlInputMax=100  Xt=0.86  Rv=150  lin_v=0  lim_v=0  K=2.4e-5 m^1.50000*kg^0.50000/s/bar^0.50000  Cmd_specify=off  Cmd_priority=High  Cmd=0  gamma_specify=off  gamma_priority=High  gamma=0  rho_specify=off  rho_priority=High  rho=0 kg/m^3  Xc_specify=off  Xc_priority=High  Xc=0  X_specify=off  X_priority=High  X=0  Y_specify=off  Y_priority=High  Y=0  CV_specify=off  CV_priority=High  CV=0
  FCV38 : simCryogenics_lib/Elements/Valve  CVmax=1.5  ControlInputMin=0  ControlInputMax=100  Xt=0.86  Rv=100  lin_v=0  lim_v=0  K=2.4e-5 m^1.50000*kg^0.50000/s/bar^0.50000  Cmd_specify=off  Cmd_priority=High  Cmd=0  gamma_specify=off  gamma_priority=High  gamma=0  rho_specify=off  rho_priority=High  rho=0 kg/m^3  Xc_specify=off  Xc_priority=High  Xc=0  X_specify=off  X_priority=High  X=0  Y_specify=off  Y_priority=High  Y=0  CV_specify=off  CV_priority=High  CV=0
  FT109 : simCryogenics_lib/Sensors/FT
  FT110 : Scope
  FT111 : Scope
  FT112 : simCryogenics_lib/Sensors/FT
  FT113 : simCryogenics_lib/Sensors/FT
  FT114 : Scope
  Gain19 : Gain  Gain=-10
  M src55 : simCryogenics_lib/Sources_Sinks/M src  M=0 kg/s
  M src56 : simCryogenics_lib/Sources_Sinks/M src  M=0 kg/s
  M src57 : simCryogenics_lib/Sources_Sinks/M src  M=0 kg/s
  Mixer27 : simCryogenics_lib/Elements/Mixer2
  Mux55 : Mux  Inputs=2
  Mux56 : Mux  Inputs=2
  Mux57 : Mux  Inputs=2
  P/T src37 : simCryogenics_lib/Sources_Sinks/P//T src  P=1.2 bar  T=4.4 K
  P/T src38 : simCryogenics_lib/Sources_Sinks/P//T src  P=1.2 bar  T=4.4 K
  PS-Simulink Converter{199..209} (11 alike) : nesl_utility/PS-Simulink Converter  PhysicalDomain=network_engine_domain  SubClassName=ps_output  LeftPortType=input  RightPortType=output  PseudoPeriodic=off  Frequencies=[]  Unit=1  AffineConversion=off
  PhaseSep19 : simCryogenics_lib/Elements/PhaseSep  Ideal1=1  DeltaT1=0.05 K  N1=10  h1=400 W/K  Ideal2=1  DeltaT2=0.05 K  N2=10  h2=400 W/K  hmax=0.870 m  S=0.0402 m^2  P0=1.25 bar  h0=50  T0=4.5 K
  Simulink-PS Converter{73..76} (4 alike) : nesl_utility/Simulink-PS Converter  PhysicalDomain=network_engine_domain  SubClassName=ps_input  LeftPortType=input  RightPortType=output  PseudoPeriodic=off  Frequencies=[]  NoiseDistribution=none  NoiseParameters=[]  Unit=1  AffineConversion=off  InputFiltering=off  SimscapeFilterOrder=1  InputFilterTimeConstant=0.001  UdotUserProvided=1
  TT73 : Scope
  TT74 : Scope
  TT75 : simCryogenics_lib/Sensors/PTT
  TT76 : Scope
  scope55 : Scope
  scope56 : Scope
  scope57 : Scope
  to_coldbox : PMIOPort  Port=1  Side=Left
  from_dewar : PMIOPort  Port=2  Side=Right
  wires:
  PS-Simulink Converter203/1 -> FT110/1
  Mux57/1 -> TT74/1
  Bias37/1 -> Gain19/1
  PS-Simulink Converter202/1 -> Mux55/2
  PS-Simulink Converter207/1 -> Mux56/2
  PS-Simulink Converter201/1 -> Mux57/2
  Mux55/1 -> TT73/1
  PS-Simulink Converter208/1 -> scope57/1, Bias37/1
  Constant56/1 -> Simulink-PS Converter76/1
  PS-Simulink Converter204/1 -> Mux56/1
  PS-Simulink Converter209/1 -> scope55/1
  PS-Simulink Converter199/1 -> FT114/1
  Constant55/1 -> Simulink-PS Converter74/1
  Gain19/1 -> Bias38/1
  Mux56/1 -> TT76/1
  PS-Simulink Converter200/1 -> Mux57/1
  PS-Simulink Converter205/1 -> FT111/1
  PS-Simulink Converter206/1 -> Mux55/1
  Constant54/1 -> Simulink-PS Converter73/1
  Bias38/1 -> scope56/1, Simulink-PS Converter75/1
  connections:
  FCV00 2 19/LConn2 -- Distributor25/RConn1
  M src57/RConn1 -- PhaseSep19/RConn3
  PS-Simulink Converter205/LConn1 -- FT113/RConn1
  Simulink-PS Converter73/RConn1 -- PhaseSep19/RConn4
  M src55/RConn1 -- PhaseSep19/RConn1
  BP_out-E38/RConn1 -- PS-Simulink Converter207/LConn1
  TT75/RConn1 -- PS-Simulink Converter206/LConn1
  PS-Simulink Converter203/LConn1 -- FT109/RConn1
  TT75/RConn2 -- PS-Simulink Converter202/LConn1
  from_dewar/RConn1 -- Distributor25/LConn1
  FCV38/LConn2 -- PhaseSep19/LConn1 -- BP_out-E37/LConn1 -- FT113/LConn1
  BP_out-E37/RConn2 -- PS-Simulink Converter200/LConn1
  BP_out-E38/RConn2 -- PS-Simulink Converter204/LConn1
  P/T src38/RConn1 -- PhaseSep19/LConn3
  PS-Simulink Converter208/LConn1 -- PhaseSep19/RConn5
  PhaseSep19/LConn2 -- P/T src37/RConn1
  FCV37/RConn1 -- Mixer27/LConn2 -- FT112/LConn1 -- BP_out-E38/LConn1
  FCV38/LConn1 -- Simulink-PS Converter76/RConn1
  PhaseSep19/RConn2 -- M src56/RConn1
  Distributor25/RConn2 -- FCV37/LConn2
  BP_out-E37/RConn1 -- PS-Simulink Converter201/LConn1
  Simulink-PS Converter74/RConn1 -- FCV00 2 19/LConn1
  Simulink-PS Converter75/RConn1 -- FCV37/LConn1
  FCV38/RConn1 -- to_coldbox/RConn1
  PS-Simulink Converter209/LConn1 -- PhaseSep19/LConn5
  PhaseSep19/LConn4 -- Mixer27/RConn1
  PS-Simulink Converter199/LConn1 -- FT112/RConn1
  FT109/LConn1 -- TT75/LConn1 -- FCV00 2 19/RConn1 -- Mixer27/LConn1

== system assemblage_19/End_Coldbox&dewar/PCqqch ==
  PI controller : simCryogenics_lib/Control/PI controller  ctrl_type=0  p_gain=-1000  i_gain=1 1/s  offset=60  sat_min=0  sat_max=100  c_PC_specify=off  c_PC_priority=None  c_PC=0  err_specify=off  err_priority=None  err=0  errDer_specify=off  errDer_priority=None  errDer=0
  PS Constant : fl_lib/Physical Signals/Sources/PS Constant  constant=0
  PS Constant1 : fl_lib/Physical Signals/Sources/PS Constant  constant=1.3
  PT : simCryogenics_lib/Sensors/PT
  PC : PMIOPort  Port=1  Side=Right
  PV : PMIOPort  Port=2  Side=Left
  connections:
  PT/LConn1 -- PV/RConn1
  PS Constant1/RConn1 -- PI controller/LConn3
  PI controller/RConn1 -- PC/RConn1
  PI controller/LConn1 -- PT/RConn1
  PS Constant/RConn1 -- PI controller/LConn2

== system assemblage_19/End_Coldbox&dewar/PCqqch1 ==
  PI controller : simCryogenics_lib/Control/PI controller  ctrl_type=0  p_gain=100  i_gain=1 1/s  offset=60  sat_min=0  sat_max=100  c_PC_specify=off  c_PC_priority=None  c_PC=0  err_specify=off  err_priority=None  err=0  errDer_specify=off  errDer_priority=None  errDer=0
  PS Constant : fl_lib/Physical Signals/Sources/PS Constant  constant=0
  PS Constant1 : fl_lib/Physical Signals/Sources/PS Constant  constant=11
  PT : simCryogenics_lib/Sensors/PT
  PC : PMIOPort  Port=1  Side=Right
  PV : PMIOPort  Port=2  Side=Left
  connections:
  PS Constant/RConn1 -- PI controller/LConn2
  PI controller/LConn1 -- PT/RConn1
  PI controller/RConn1 -- PC/RConn1
  PS Constant1/RConn1 -- PI controller/LConn3
  PT/LConn1 -- PV/RConn1

== system assemblage_19/End_Coldbox&dewar/Subsystem ==
  PS Add : fl_lib/Physical Signals/Functions/PS Add
  PS Gain : fl_lib/Physical Signals/Functions/PS Gain  gain=85
  PS Subtract : fl_lib/Physical Signals/Functions/PS Subtract
  pression_3b : fl_lib/Physical Signals/Sources/PS Constant  constant=3
  "vanne_63 " : fl_lib/Physical Signals/Sources/PS Constant  constant=63
  PV : PMIOPort  Port=1  Side=Right
  PC : PMIOPort  Port=2  Side=Left
  connections:
  pression_3b/RConn1 -- PS Subtract/LConn2
  PS Subtract/RConn1 -- PS Gain/LConn1
  PS Gain/RConn1 -- PS Add/LConn1
  PS Subtract/LConn1 -- PV/RConn1
  "vanne_63 "/RConn1 -- PS Add/LConn2
  PS Add/RConn1 -- PC/RConn1
